simulink model "Dpt_S_Fun_1_M"  (Simulink 4.00)
settings: Solver=ode45  SolverMode=SingleTasking  StartTime=0.0  StopTime=0.4  MaxStep=0.001  RelTol=1e-3  AbsTol=1e-3
PreLoadFcn:
  | Load_Param_1
values from neighbouring files (symbols this model uses):
  Cm = 10    [Load_Param_1.m]
  Cw = 10    [Load_Param_1.m]
  Fi = 1    [Load_Param_1.m]
  J = 10    [Load_Param_1.m]
  L = 0.001    [Load_Param_1.m]
  Mnabr = 2500    [Load_Param_1.m]
  R = 0.1    [Load_Param_1.m]
  Tnabr = 0.2    [Load_Param_1.m]
  V = 220    [Load_Param_1.m]
settings Model: LastModifiedBy=Администратор  SaveTime=off  SaveOutput=off  LimitDataPoints=off  RTWTemplateMakefile=grt_vc.tmf  BlockReductionOpt=off

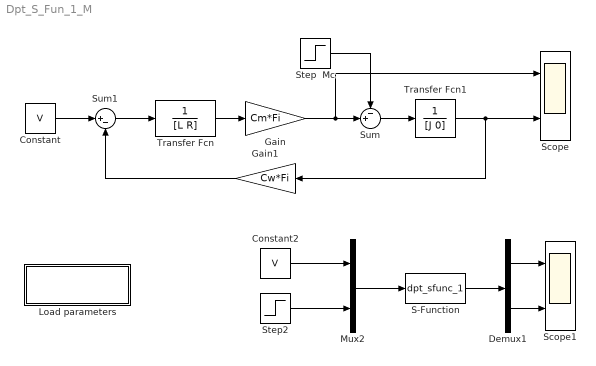
== system Dpt_S_Fun_1_M ==
  Constant : Constant  Value=V
  Constant2 : Constant  Value=V
  Demux1 : Demux  Outputs=2  BusSelectionMode=off
  Gain : Gain  Gain=Cm*Fi  Multiplication=Element-wise(K.*u)  SaturateOnIntegerOverflow=on
  Gain1 : Gain  Orientation=left  Gain=Cw*Fi  Multiplication=Element-wise(K.*u)  SaturateOnIntegerOverflow=on
  Load parameters : Subsystem
      settings: OpenFcn=Load_Param_1  RTWFcnNameOpts=Auto  RTWFileNameOpts=Auto
      mask Help: Click here to save t and yout in an ascii data file called temp.dat
      mask Display: disp('Click here to\n load parameters')
  Mux2 : Mux  Inputs=2
  S-Function : S-Function  FunctionName=dpt_sfunc_1  Parameters=L,R,J,Cm,Cw,Fi  PortCounts=[]  SFunctionModules=''
  Scope : Scope  NumInputPorts=2
      settings: TimeRange=0.4  YMin=-3286.73~0  YMax=12937.8~30  SaveToWorkspace=off  SaveName=ScopeData  LimitDataPoints=on  MaxDataPoints=5000
  Scope1 : Scope  NumInputPorts=2
      settings: TimeRange=0.4  YMin=-3286.73~0  YMax=12937.8~30  SaveToWorkspace=off  LimitDataPoints=on  MaxDataPoints=5000
  Step  Mc : Step  Time=Tnabr  Before=0  After=Mnabr  SampleTime=0
  Step2 : Step  Time=Tnabr  Before=0  After=Mnabr  SampleTime=0
  Sum : Sum  Inputs=-+|  SaturateOnIntegerOverflow=on
  Sum1 : Sum  Inputs=|+-  SaturateOnIntegerOverflow=on
  Transfer Fcn : TransferFcn  Numerator=[1]  Denominator=[L R]  AbsoluteTolerance=auto  Realization=auto
  Transfer Fcn1 : TransferFcn  Numerator=[1]  Denominator=[J 0]  AbsoluteTolerance=auto  Realization=auto
  wires:
  Constant/1 -> Sum1/1
  Sum1/1 -> Transfer Fcn/1
  Step  Mc/1 -> Sum/1
  Sum/1 -> Transfer Fcn1/1
  Transfer Fcn/1 -> Gain/1
  Gain/1 -> Sum/2, Scope/1
  Transfer Fcn1/1 -> Gain1/1, Scope/2
  Gain1/1 -> Sum1/2
  Constant2/1 -> Mux2/1
  Step2/1 -> Mux2/2
  Mux2/1 -> S-Function/1
  Demux1/1 -> Scope1/1
  Demux1/2 -> Scope1/2
  S-Function/1 -> Demux1/1

== system Dpt_S_Fun_1_M/Load parameters ==
  note: a
